simulink model "Codex_sim"  (R2023b)
settings: Solver=VariableStepAuto  StartTime=0.0  StopTime=10  RelTol=1e-3
values from neighbouring files (symbols this model uses):
  A_val = cell(1,3)    [codex.m]
  B_val = cell(1,3)    [codex.m]
  C = [0 1]    [codex.m]
  K_val = cell(1,3)    [codex.m]
undefined symbols (not defined in the file or in its folder): B1, J1, Kb1, Kt1, L1, R1
libraries: spspowerguiLib x1
settings Model: Creator=Hi  LastModifiedBy=Hi

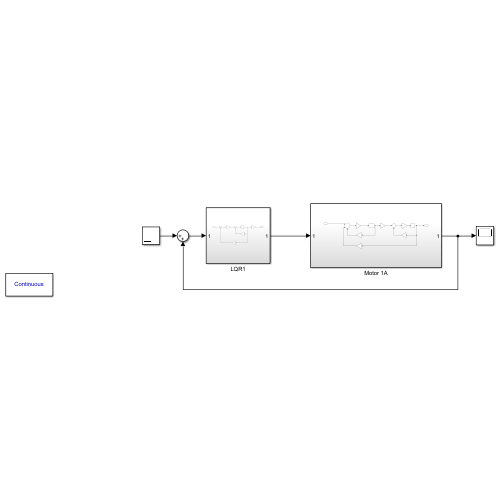
[thumbnail: Simulink's stored preview of the top-level diagram]
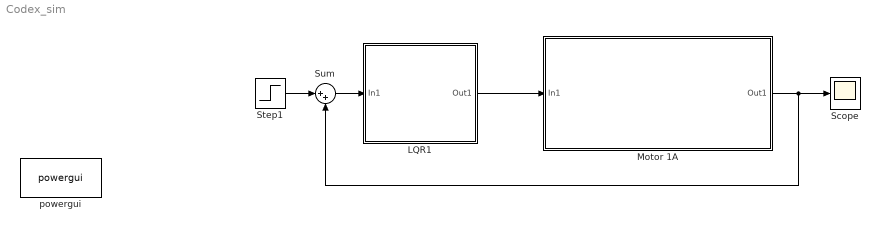
== system Codex_sim ==
  LQR1 : Subsystem
  Motor 1A : Subsystem
  Scope : Scope
  Step1 : Step  Time=0.00001  SampleTime=0
  Sum : Sum  Inputs=|++
  powergui : spspowerguiLib/powergui  Priority=1  SimulationMode=Continuous  SampleTime=50e-6  frequency=60  Iterations=50  frequencyindice=60  Pbase=100e6  ErrMax=1e-4  UnitsV=kV  UnitsW=MW  buscounter=0  FunctionMessages=off  echomessages=off  EnableUseOfTLC=off  CurrentSourceSwitches=off  DisableSnubberDevices=off  DisableRonSwitches=off  DisableVfSwitches=off  DisplayEquations=off  AutomaticDiscreteSolvers=off  SolverType=Tustin/Backward Euler (TBE)  Interpol=off  ExternalGateDelay=off  methode=off  Ts=100  x0status=blocks  SPID=on  SwTol=0  HookPort=off  NonlinearTolerance=1e-4  nMaxIteration=100  ContinueOnMaxIteration=off  RestoreLinks=warning  ResistiveCurrentMeasurement=off  Frange=[0:2:500]  Ylog=off  Xlog=on  ShowGrid=off  save=off  variable=ZData  structure=0  ZoomFFT=off  StartTime=0.0  cycles=1  DisplayStyle=1  fundamental=60  FreqAxis=off  MaxFrequency=1000  frequencyindicesteady=1  RmsSteady=1  display=off
  wires:
  LQR1/1(Out1) -> Motor 1A/1(In1)
  Motor 1A/1(Out1) -> Sum/2, Scope/1
  Step1/1 -> Sum/1
  Sum/1 -> LQR1/1(In1)

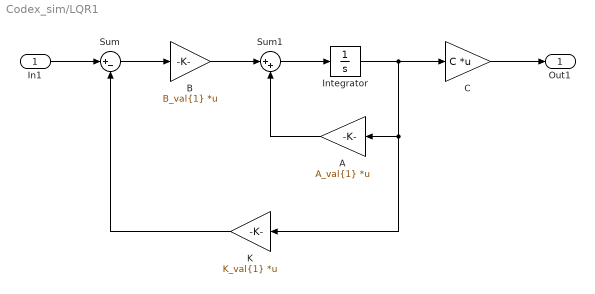
== system Codex_sim/LQR1 ==
  In1 : Inport
  A : Gain  Gain=A_val{1}  Multiplication=Matrix(K*u)
  B : Gain  Gain=B_val{1}  Multiplication=Matrix(K*u)
  C : Gain  Gain=C  Multiplication=Matrix(K*u)
  Integrator : Integrator
  K : Gain  Gain=K_val{1}  Multiplication=Matrix(K*u)
  Sum : Sum  Inputs=|+-
  Sum1 : Sum  Inputs=|++
  Out1 : Outport
  wires:
  C/1 -> Out1/1
  Sum/1 -> B/1
  Sum1/1 -> Integrator/1
  K/1 -> Sum/2
  Integrator/1 -> K/1, A/1, C/1
  B/1 -> Sum1/1
  In1/1 -> Sum/1
  A/1 -> Sum1/2

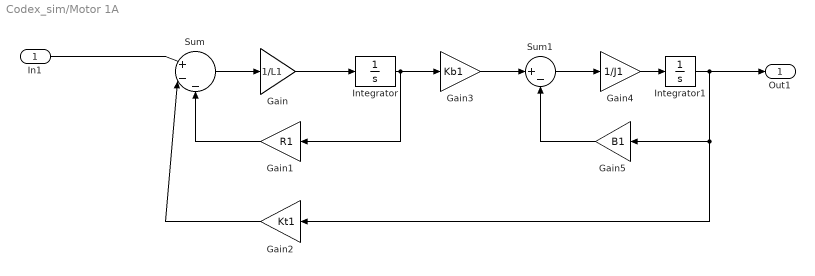
== system Codex_sim/Motor 1A ==
  In1 : Inport
  Gain : Gain  Gain=1/L1
  Gain1 : Gain  Gain=R1
  Gain2 : Gain  Gain=Kt1
  Gain3 : Gain  Gain=Kb1
  Gain4 : Gain  Gain=1/J1
  Gain5 : Gain  Gain=B1
  Integrator : Integrator
  Integrator1 : Integrator
  Sum : Sum  Inputs=|+--  OutDataTypeStr=Inherit: Keep LSB
  Sum1 : Sum  Inputs=|+-
  Out1 : Outport
  wires:
  Gain2/1 -> Sum/2
  Gain/1 -> Integrator/1
  Gain4/1 -> Integrator1/1
  Integrator/1 -> Gain1/1, Gain3/1
  Gain1/1 -> Sum/3
  Gain3/1 -> Sum1/1
  Gain5/1 -> Sum1/2
  Sum/1 -> Gain/1
  Sum1/1 -> Gain4/1
  In1/1 -> Sum/1
  Integrator1/1 -> Out1/1, Gain5/1, Gain2/1
